simulink model "blending_tank_auto"  (R2020b)
settings: Solver=FixedStepAuto  StartTime=0.0  StopTime=Inf  RelTol=1e-3
PostLoadFcn:
  | slplc.api.loadDataTypes;
InitFcn:
  | T1_InitialValue = FB_TON.InitialValue;
  | T1_InitialValue.PRE = 20000;
  | 
  | C1_InitialValue = FB_CTU.InitialValue;
  | C1_InitialValue.PRE = 3;
StopFcn:
  | clear T1_InitialValue C1_InitialValue;
undefined symbols (not defined in the file): BOOL, DINT, OTL, REAL, slplc
libraries: simulink x3, sldrtlib x1
(part 2 of 15)

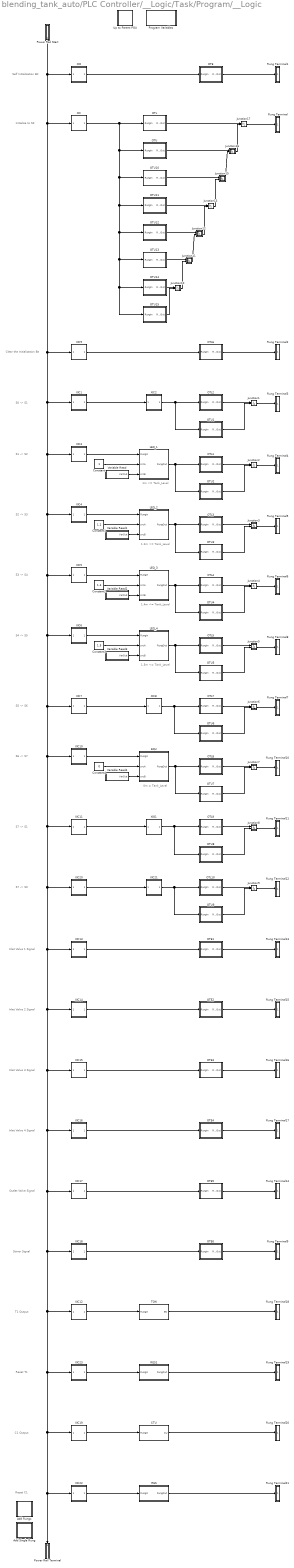
== system blending_tank_auto/PLC Controller/__Logic/Task/Program/__Logic ==
  note: Clear the Initialisation Bit
  note: Self Initialisation Bit
  note: Initialise to S0
  note: S1 -> S2
  note: S0 -> S1
  note: S6 -> S7
  note: S7 -> S1
  note: Inlet Valve 1 Signal
  note: Inlet Valve 2 Signal
  note: Inlet Valve 3 Signal
  note: Inlet Valve 4 Signal
  note: Outlet Valve Signal
  note: Stirrer Signal
  note: S2 -> S3
  note: S3 -> S4
  note: S5 -> S6
  note: S4 -> S5
  note: T1 Output
  note: C1 Output
  note: S7 -> S0
  note: Reset T1
  note: Reset C1
  note: 1m <= Tank_Level
  note: 1.2m <= Tank_Level
  note: 1.4m <= Tank_Level
  note: 1.5m <= Tank_Level
  note: 0m = Tank_Level
  Add Rungs : Subsystem  DisableCoverage=on  TreatAsAtomicUnit=on  mask{PLCRungNumberToAdd=18, PLCBlockType=AddRungs}
      mask prompts: PLCRungNumberToAdd "Rung Number:"
      mask Help: web([docroot '/plccoder/ref/addrungs' '.html']);
      mask DialogControl PLCAddRungs Prompt: Add Rungs
      mask DialogControl PLCRungAddButton Prompt: Add
      mask DialogControl PLCRungAddButton Callback: slplc.callbacks.addLadderRungs(gcb);
      mask Display: disp(sprintf(['Add' newline 'Rungs']));
  Add Single Rung : Subsystem  DisableCoverage=on  TreatAsAtomicUnit=on  mask{PLCRungNumberToAdd=1, PLCBlockType=AddSingleRung}
      settings: OpenFcn=slplc.callbacks.addLadderRungs(gcb);
      mask Help: web([docroot '/plccoder/ref/addsinglerung' '.html']);
      mask DialogControl PLCAddRung Prompt: Add Single Rung
      mask Display: disp(sprintf(['Add' newline '1 Rung']));
  CTU : Subsystem  Priority=114  TreatAsAtomicUnit=on  mask{PLCOperandTag=C1, PLCBlockType=CTU, PLCPOUType=stdFB, PLCOperandAccess=ReadWrite, PLCOperandExpression=xxx_PLC_VAR_C1}
      mask prompts: PLCOperandTag "Counter Tag:"
      mask init:
      | block = gcb;
      | maskObj = Simulink.Mask.get(block);
      | maskObj.Display = sprintf('disp([''%s'' newline newline ''%s'']);', 'CTU', PLCOperandTag);
      | slplc.callbacks.initInstruction(block);
      settings: AttributesFormatString=%<PLCBlockType>: %<PLCOperandTag>
      mask Help: web([docroot '/plccoder/ref/ctu' '.html']);
      mask DialogControl PLCBlockTitle Prompt: Count Up (CTU)
      mask Display: disp(['CTU' newline newline 'C1']);
  Constant : Constant  Priority=32  OutDataTypeStr=double
  Constant1 : Constant  Priority=40  Value=1.2  OutDataTypeStr=double
  Constant2 : Constant  Priority=48  Value=1.4  OutDataTypeStr=double
  Constant3 : Constant  Priority=56  Value=1.5  OutDataTypeStr=double
  Constant4 : Constant  Priority=70  Value=0  OutDataTypeStr=double
  EQU : Subsystem  Priority=72  TreatAsAtomicUnit=on  mask{PLCBlockType=EQU, PLCPOUType=stdFC}
      mask Help: web([docroot '/plccoder/ref/equ' '.html']);
      mask DialogControl PLCBlockTitle Prompt: Equal To (EQU)
      mask DialogControl PLCBlockDesc Prompt: Test whether Source A is equal to Source B.
      mask Display: disp('EQU');
  Junction1 : Subsystem  Priority=29  DisableCoverage=on  TreatAsAtomicUnit=on  mask{PLCBlockType=Junction, PLCPOUType=BranchJunction}
      mask Help: web([docroot '/plccoder/ref/junction' '.html']);
      mask DialogControl PLCBlockTitle Prompt: Rung Merge Point
      mask DialogControl PLCBlockDesc Prompt: This is the ladder diagram rung merge point.
  Junction10 : Subsystem  Priority=14  DisableCoverage=on  TreatAsAtomicUnit=on  mask{PLCBlockType=Junction, PLCPOUType=BranchJunction}
      mask Help: web([docroot '/plccoder/ref/junction' '.html']);
      mask DialogControl PLCBlockTitle Prompt: Rung Merge Point
      mask DialogControl PLCBlockDesc Prompt: This is the ladder diagram rung merge point.
  Junction11 : Subsystem  Priority=15  DisableCoverage=on  TreatAsAtomicUnit=on  mask{PLCBlockType=Junction, PLCPOUType=BranchJunction}
      mask Help: web([docroot '/plccoder/ref/junction' '.html']);
      mask DialogControl PLCBlockTitle Prompt: Rung Merge Point
      mask DialogControl PLCBlockDesc Prompt: This is the ladder diagram rung merge point.
  Junction12 : Subsystem  Priority=16  DisableCoverage=on  TreatAsAtomicUnit=on  mask{PLCBlockType=Junction, PLCPOUType=BranchJunction}
      mask Help: web([docroot '/plccoder/ref/junction' '.html']);
      mask DialogControl PLCBlockTitle Prompt: Rung Merge Point
      mask DialogControl PLCBlockDesc Prompt: This is the ladder diagram rung merge point.
  Junction13 : Subsystem  Priority=17  DisableCoverage=on  TreatAsAtomicUnit=on  mask{PLCBlockType=Junction, PLCPOUType=BranchJunction}
      mask Help: web([docroot '/plccoder/ref/junction' '.html']);
      mask DialogControl PLCBlockTitle Prompt: Rung Merge Point
      mask DialogControl PLCBlockDesc Prompt: This is the ladder diagram rung merge point.
  Junction15 : Subsystem  Priority=18  DisableCoverage=on  TreatAsAtomicUnit=on  mask{PLCBlockType=Junction, PLCPOUType=BranchJunction}
      mask Help: web([docroot '/plccoder/ref/junction' '.html']);
      mask DialogControl PLCBlockTitle Prompt: Rung Merge Point
      mask DialogControl PLCBlockDesc Prompt: This is the ladder diagram rung merge point.
  Junction16 : Subsystem  Priority=19  DisableCoverage=on  TreatAsAtomicUnit=on  mask{PLCBlockType=Junction, PLCPOUType=BranchJunction}
      mask Help: web([docroot '/plccoder/ref/junction' '.html']);
      mask DialogControl PLCBlockTitle Prompt: Rung Merge Point
      mask DialogControl PLCBlockDesc Prompt: This is the ladder diagram rung merge point.
  Junction17 : Subsystem  Priority=20  DisableCoverage=on  TreatAsAtomicUnit=on  mask{PLCBlockType=Junction, PLCPOUType=BranchJunction}
      mask Help: web([docroot '/plccoder/ref/junction' '.html']);
      mask DialogControl PLCBlockTitle Prompt: Rung Merge Point
      mask DialogControl PLCBlockDesc Prompt: This is the ladder diagram rung merge point.
  Junction2 : Subsystem  Priority=37  DisableCoverage=on  TreatAsAtomicUnit=on  mask{PLCBlockType=Junction, PLCPOUType=BranchJunction}
      mask Help: web([docroot '/plccoder/ref/junction' '.html']);
      mask DialogControl PLCBlockTitle Prompt: Rung Merge Point
      mask DialogControl PLCBlockDesc Prompt: This is the ladder diagram rung merge point.
  Junction3 : Subsystem  Priority=45  DisableCoverage=on  TreatAsAtomicUnit=on  mask{PLCBlockType=Junction, PLCPOUType=BranchJunction}
      mask Help: web([docroot '/plccoder/ref/junction' '.html']);
      mask DialogControl PLCBlockTitle Prompt: Rung Merge Point
      mask DialogControl PLCBlockDesc Prompt: This is the ladder diagram rung merge point.
  Junction4 : Subsystem  Priority=53  DisableCoverage=on  TreatAsAtomicUnit=on  mask{PLCBlockType=Junction, PLCPOUType=BranchJunction}
      mask Help: web([docroot '/plccoder/ref/junction' '.html']);
      mask DialogControl PLCBlockTitle Prompt: Rung Merge Point
      mask DialogControl PLCBlockDesc Prompt: This is the ladder diagram rung merge point.
  Junction5 : Subsystem  Priority=61  DisableCoverage=on  TreatAsAtomicUnit=on  mask{PLCBlockType=Junction, PLCPOUType=BranchJunction}
      mask Help: web([docroot '/plccoder/ref/junction' '.html']);
      mask DialogControl PLCBlockTitle Prompt: Rung Merge Point
      mask DialogControl PLCBlockDesc Prompt: This is the ladder diagram rung merge point.
  Junction6 : Subsystem  Priority=67  DisableCoverage=on  TreatAsAtomicUnit=on  mask{PLCBlockType=Junction, PLCPOUType=BranchJunction}
      mask Help: web([docroot '/plccoder/ref/junction' '.html']);
      mask DialogControl PLCBlockTitle Prompt: Rung Merge Point
      mask DialogControl PLCBlockDesc Prompt: This is the ladder diagram rung merge point.
  Junction7 : Subsystem  Priority=75  DisableCoverage=on  TreatAsAtomicUnit=on  mask{PLCBlockType=Junction, PLCPOUType=BranchJunction}
      mask Help: web([docroot '/plccoder/ref/junction' '.html']);
      mask DialogControl PLCBlockTitle Prompt: Rung Merge Point
      mask DialogControl PLCBlockDesc Prompt: This is the ladder diagram rung merge point.
  Junction8 : Subsystem  Priority=81  DisableCoverage=on  TreatAsAtomicUnit=on  mask{PLCBlockType=Junction, PLCPOUType=BranchJunction}
      mask Help: web([docroot '/plccoder/ref/junction' '.html']);
      mask DialogControl PLCBlockTitle Prompt: Rung Merge Point
      mask DialogControl PLCBlockDesc Prompt: This is the ladder diagram rung merge point.
  Junction9 : Subsystem  Priority=87  DisableCoverage=on  TreatAsAtomicUnit=on  mask{PLCBlockType=Junction, PLCPOUType=BranchJunction}
      mask Help: web([docroot '/plccoder/ref/junction' '.html']);
      mask DialogControl PLCBlockTitle Prompt: Rung Merge Point
      mask DialogControl PLCBlockDesc Prompt: This is the ladder diagram rung merge point.
  LEQ_1 : Subsystem  Priority=34  TreatAsAtomicUnit=on  mask{PLCBlockType=LEQ, PLCPOUType=stdFC}
      mask Help: web([docroot '/plccoder/ref/leq' '.html']);
      mask DialogControl PLCBlockTitle Prompt: Less Than or Equal To (LEQ)
      mask DialogControl PLCBlockDesc Prompt: Test whether Source A is less than or equal to Source B.
      mask Display: disp('LEQ');
  LEQ_2 : Subsystem  Priority=42  TreatAsAtomicUnit=on  mask{PLCBlockType=LEQ, PLCPOUType=stdFC}
      mask Help: web([docroot '/plccoder/ref/leq' '.html']);
      mask DialogControl PLCBlockTitle Prompt: Less Than or Equal To (LEQ)
      mask DialogControl PLCBlockDesc Prompt: Test whether Source A is less than or equal to Source B.
      mask Display: disp('LEQ');
  LEQ_3 : Subsystem  Priority=50  TreatAsAtomicUnit=on  mask{PLCBlockType=LEQ, PLCPOUType=stdFC}
      mask Help: web([docroot '/plccoder/ref/leq' '.html']);
      mask DialogControl PLCBlockTitle Prompt: Less Than or Equal To (LEQ)
      mask DialogControl PLCBlockDesc Prompt: Test whether Source A is less than or equal to Source B.
      mask Display: disp('LEQ');
  LEQ_4 : Subsystem  Priority=58  TreatAsAtomicUnit=on  mask{PLCBlockType=LEQ, PLCPOUType=stdFC}
      mask Help: web([docroot '/plccoder/ref/leq' '.html']);
      mask DialogControl PLCBlockTitle Prompt: Less Than or Equal To (LEQ)
      mask DialogControl PLCBlockDesc Prompt: Test whether Source A is less than or equal to Source B.
      mask Display: disp('LEQ');
  OTE : Subsystem  Priority=3  TreatAsAtomicUnit=on  mask{PLCOperandTag=Initialise, PLCBlockType=OTE, PLCPOUType=Coil, PLCOperandExpression=xxx_PLC_VAR_Initialise}
      mask prompts: PLCOperandTag "Operand Tag:"
      mask init:
      | slplc.callbacks.initInstruction(gcb);
      settings: AttributesFormatString=%<PLCOperandTag>
      mask Help: web([docroot '/plccoder/ref/ote' '.html']);
      mask DialogControl PLCBlockTitle Prompt: Output Energize (OTE)
  OTE1 : Subsystem  Priority=90  TreatAsAtomicUnit=on  mask{PLCOperandTag=IV1_Signal, PLCBlockType=OTE, PLCPOUType=Coil, PLCOperandExpression=xxx_PLC_VAR_IV1_Signal}
      mask prompts: PLCOperandTag "Operand Tag:"
      mask init:
      | slplc.callbacks.initInstruction(gcb);
      settings: AttributesFormatString=%<PLCOperandTag>
      mask Help: web([docroot '/plccoder/ref/ote' '.html']);
      mask DialogControl PLCBlockTitle Prompt: Output Energize (OTE)
  OTE2 : Subsystem  Priority=93  TreatAsAtomicUnit=on  mask{PLCOperandTag=IV2_Signal, PLCBlockType=OTE, PLCPOUType=Coil, PLCOperandExpression=xxx_PLC_VAR_IV2_Signal}
      mask prompts: PLCOperandTag "Operand Tag:"
      mask init:
      | slplc.callbacks.initInstruction(gcb);
      settings: AttributesFormatString=%<PLCOperandTag>
      mask Help: web([docroot '/plccoder/ref/ote' '.html']);
      mask DialogControl PLCBlockTitle Prompt: Output Energize (OTE)
  OTE3 : Subsystem  Priority=96  TreatAsAtomicUnit=on  mask{PLCOperandTag=IV3_Signal, PLCBlockType=OTE, PLCPOUType=Coil, PLCOperandExpression=xxx_PLC_VAR_IV3_Signal}
      mask prompts: PLCOperandTag "Operand Tag:"
      mask init:
      | slplc.callbacks.initInstruction(gcb);
      settings: AttributesFormatString=%<PLCOperandTag>
      mask Help: web([docroot '/plccoder/ref/ote' '.html']);
      mask DialogControl PLCBlockTitle Prompt: Output Energize (OTE)
  OTE4 : Subsystem  Priority=99  TreatAsAtomicUnit=on  mask{PLCOperandTag=IV4_Signal, PLCBlockType=OTE, PLCPOUType=Coil, PLCOperandExpression=xxx_PLC_VAR_IV4_Signal}
      mask prompts: PLCOperandTag "Operand Tag:"
      mask init:
      | slplc.callbacks.initInstruction(gcb);
      settings: AttributesFormatString=%<PLCOperandTag>
      mask Help: web([docroot '/plccoder/ref/ote' '.html']);
      mask DialogControl PLCBlockTitle Prompt: Output Energize (OTE)
  OTE5 : Subsystem  Priority=102  TreatAsAtomicUnit=on  mask{PLCOperandTag=OV_Signal, PLCBlockType=OTE, PLCPOUType=Coil, PLCOperandExpression=xxx_PLC_VAR_OV_Signal}
      mask prompts: PLCOperandTag "Operand Tag:"
      mask init:
      | slplc.callbacks.initInstruction(gcb);
      settings: AttributesFormatString=%<PLCOperandTag>
      mask Help: web([docroot '/plccoder/ref/ote' '.html']);
      mask DialogControl PLCBlockTitle Prompt: Output Energize (OTE)
  OTE6 : Subsystem  Priority=105  TreatAsAtomicUnit=on  mask{PLCOperandTag=Stirrer_Signal, PLCBlockType=OTE, PLCPOUType=Coil, PLCOperandExpression=xxx_PLC_VAR_Stirrer_Signal}
      mask prompts: PLCOperandTag "Operand Tag:"
      mask init:
      | slplc.callbacks.initInstruction(gcb);
      settings: AttributesFormatString=%<PLCOperandTag>
      mask Help: web([docroot '/plccoder/ref/ote' '.html']);
      mask DialogControl PLCBlockTitle Prompt: Output Energize (OTE)
  OTL : Subsystem  Priority=6  TreatAsAtomicUnit=on  mask{PLCOperandTag=M0, PLCBlockType=OTL, PLCPOUType=Coil, PLCOperandExpression=xxx_PLC_VAR_M0}
      mask prompts: PLCOperandTag "Operand Tag:"
      mask init:
      | slplc.callbacks.initInstruction(gcb);
      settings: AttributesFormatString=%<PLCOperandTag>
      mask Help: web([docroot '/plccoder/ref/otl' '.html']);
      mask DialogControl PLCBlockTitle Prompt: Output Latch (OTL)
      mask Display: disp('L');
  OTL1 : Subsystem  Priority=35  TreatAsAtomicUnit=on  mask{PLCOperandTag=M2, PLCBlockType=OTL, PLCPOUType=Coil, PLCOperandExpression=xxx_PLC_VAR_M2}
      mask prompts: PLCOperandTag "Operand Tag:"
      mask init:
      | slplc.callbacks.initInstruction(gcb);
      settings: AttributesFormatString=%<PLCOperandTag>
      mask Help: web([docroot '/plccoder/ref/otl' '.html']);
      mask DialogControl PLCBlockTitle Prompt: Output Latch (OTL)
      mask Display: disp('L');
  OTL10 : Subsystem  Priority=85  TreatAsAtomicUnit=on  mask{PLCOperandTag=M0, PLCBlockType=OTL, PLCPOUType=Coil, PLCOperandExpression=xxx_PLC_VAR_M0}
      mask prompts: PLCOperandTag "Operand Tag:"
      mask init:
      | slplc.callbacks.initInstruction(gcb);
      settings: AttributesFormatString=%<PLCOperandTag>
      mask Help: web([docroot '/plccoder/ref/otl' '.html']);
      mask DialogControl PLCBlockTitle Prompt: Output Latch (OTL)
      mask Display: disp('L');
  OTL2 : Subsystem  Priority=27  TreatAsAtomicUnit=on  mask{PLCOperandTag=M1, PLCBlockType=OTL, PLCPOUType=Coil, PLCOperandExpression=xxx_PLC_VAR_M1}
      mask prompts: PLCOperandTag "Operand Tag:"
      mask init:
      | slplc.callbacks.initInstruction(gcb);
      settings: AttributesFormatString=%<PLCOperandTag>
      mask Help: web([docroot '/plccoder/ref/otl' '.html']);
      mask DialogControl PLCBlockTitle Prompt: Output Latch (OTL)
      mask Display: disp('L');
  OTL3 : Subsystem  Priority=43  TreatAsAtomicUnit=on  mask{PLCOperandTag=M3, PLCBlockType=OTL, PLCPOUType=Coil, PLCOperandExpression=xxx_PLC_VAR_M3}
      mask prompts: PLCOperandTag "Operand Tag:"
      mask init:
      | slplc.callbacks.initInstruction(gcb);
      settings: AttributesFormatString=%<PLCOperandTag>
      mask Help: web([docroot '/plccoder/ref/otl' '.html']);
      mask DialogControl PLCBlockTitle Prompt: Output Latch (OTL)
      mask Display: disp('L');
  OTL4 : Subsystem  Priority=51  TreatAsAtomicUnit=on  mask{PLCOperandTag=M4, PLCBlockType=OTL, PLCPOUType=Coil, PLCOperandExpression=xxx_PLC_VAR_M4}
      mask prompts: PLCOperandTag "Operand Tag:"
      mask init:
      | slplc.callbacks.initInstruction(gcb);
      settings: AttributesFormatString=%<PLCOperandTag>
      mask Help: web([docroot '/plccoder/ref/otl' '.html']);
      mask DialogControl PLCBlockTitle Prompt: Output Latch (OTL)
      mask Display: disp('L');
  OTL5 : Subsystem  Priority=59  TreatAsAtomicUnit=on  mask{PLCOperandTag=M5, PLCBlockType=OTL, PLCPOUType=Coil, PLCOperandExpression=xxx_PLC_VAR_M5}
      mask prompts: PLCOperandTag "Operand Tag:"
      mask init:
      | slplc.callbacks.initInstruction(gcb);
      settings: AttributesFormatString=%<PLCOperandTag>
      mask Help: web([docroot '/plccoder/ref/otl' '.html']);
      mask DialogControl PLCBlockTitle Prompt: Output Latch (OTL)
      mask Display: disp('L');
  OTL6 : Subsystem  Priority=23  TreatAsAtomicUnit=on  mask{PLCOperandTag=Running, PLCBlockType=OTL, PLCPOUType=Coil, PLCOperandExpression=xxx_PLC_VAR_Running}
      mask prompts: PLCOperandTag "Operand Tag:"
      mask init:
      | slplc.callbacks.initInstruction(gcb);
      settings: AttributesFormatString=%<PLCOperandTag>
      mask Help: web([docroot '/plccoder/ref/otl' '.html']);
      mask DialogControl PLCBlockTitle Prompt: Output Latch (OTL)
      mask Display: disp('L');
  OTL7 : Subsystem  Priority=65  TreatAsAtomicUnit=on  mask{PLCOperandTag=M6, PLCBlockType=OTL, PLCPOUType=Coil, PLCOperandExpression=xxx_PLC_VAR_M6}
      mask prompts: PLCOperandTag "Operand Tag:"
      mask init:
      | slplc.callbacks.initInstruction(gcb);
      settings: AttributesFormatString=%<PLCOperandTag>
      mask Help: web([docroot '/plccoder/ref/otl' '.html']);
      mask DialogControl PLCBlockTitle Prompt: Output Latch (OTL)
      mask Display: disp('L');
  OTL8 : Subsystem  Priority=73  TreatAsAtomicUnit=on  mask{PLCOperandTag=M7, PLCBlockType=OTL, PLCPOUType=Coil, PLCOperandExpression=xxx_PLC_VAR_M7}
      mask prompts: PLCOperandTag "Operand Tag:"
      mask init:
      | slplc.callbacks.initInstruction(gcb);
      settings: AttributesFormatString=%<PLCOperandTag>
      mask Help: web([docroot '/plccoder/ref/otl' '.html']);
      mask DialogControl PLCBlockTitle Prompt: Output Latch (OTL)
      mask Display: disp('L');
  OTL9 : Subsystem  Priority=79  TreatAsAtomicUnit=on  mask{PLCOperandTag=M1, PLCBlockType=OTL, PLCPOUType=Coil, PLCOperandExpression=xxx_PLC_VAR_M1}
      mask prompts: PLCOperandTag "Operand Tag:"
      mask init:
      | slplc.callbacks.initInstruction(gcb);
      settings: AttributesFormatString=%<PLCOperandTag>
      mask Help: web([docroot '/plccoder/ref/otl' '.html']);
      mask DialogControl PLCBlockTitle Prompt: Output Latch (OTL)
      mask Display: disp('L');
  OTU : Subsystem  Priority=7  TreatAsAtomicUnit=on  mask{PLCOperandTag=M1, PLCBlockType=OTU, PLCPOUType=Coil, PLCOperandExpression=xxx_PLC_VAR_M1}
      mask prompts: PLCOperandTag "Operand Tag:"
      mask init:
      | slplc.callbacks.initInstruction(gcb);
      settings: AttributesFormatString=%<PLCOperandTag>
      mask Help: web([docroot '/plccoder/ref/otu' '.html']);
      mask DialogControl PLCBlockTitle Prompt: Output Unlatch (OTU)
      mask Display: disp('U');
  OTU1 : Subsystem  Priority=28  TreatAsAtomicUnit=on  mask{PLCOperandTag=M0, PLCBlockType=OTU, PLCPOUType=Coil, PLCOperandExpression=xxx_PLC_VAR_M0}
      mask prompts: PLCOperandTag "Operand Tag:"
      mask init:
      | slplc.callbacks.initInstruction(gcb);
      settings: AttributesFormatString=%<PLCOperandTag>
      mask Help: web([docroot '/plccoder/ref/otu' '.html']);
      mask DialogControl PLCBlockTitle Prompt: Output Unlatch (OTU)
      mask Display: disp('U');
  OTU10 : Subsystem  Priority=8  TreatAsAtomicUnit=on  mask{PLCOperandTag=M2, PLCBlockType=OTU, PLCPOUType=Coil, PLCOperandExpression=xxx_PLC_VAR_M2}
      mask prompts: PLCOperandTag "Operand Tag:"
      mask init:
      | slplc.callbacks.initInstruction(gcb);
      settings: AttributesFormatString=%<PLCOperandTag>
      mask Help: web([docroot '/plccoder/ref/otu' '.html']);
      mask DialogControl PLCBlockTitle Prompt: Output Unlatch (OTU)
      mask Display: disp('U');
  OTU11 : Subsystem  Priority=9  TreatAsAtomicUnit=on  mask{PLCOperandTag=M3, PLCBlockType=OTU, PLCPOUType=Coil, PLCOperandExpression=xxx_PLC_VAR_M3}
      mask prompts: PLCOperandTag "Operand Tag:"
      mask init:
      | slplc.callbacks.initInstruction(gcb);
      settings: AttributesFormatString=%<PLCOperandTag>
      mask Help: web([docroot '/plccoder/ref/otu' '.html']);
      mask DialogControl PLCBlockTitle Prompt: Output Unlatch (OTU)
      mask Display: disp('U');
  OTU12 : Subsystem  Priority=10  TreatAsAtomicUnit=on  mask{PLCOperandTag=M4, PLCBlockType=OTU, PLCPOUType=Coil, PLCOperandExpression=xxx_PLC_VAR_M4}
      mask prompts: PLCOperandTag "Operand Tag:"
      mask init:
      | slplc.callbacks.initInstruction(gcb);
      settings: AttributesFormatString=%<PLCOperandTag>
      mask Help: web([docroot '/plccoder/ref/otu' '.html']);
      mask DialogControl PLCBlockTitle Prompt: Output Unlatch (OTU)
      mask Display: disp('U');
  OTU13 : Subsystem  Priority=11  TreatAsAtomicUnit=on  mask{PLCOperandTag=M5, PLCBlockType=OTU, PLCPOUType=Coil, PLCOperandExpression=xxx_PLC_VAR_M5}
      mask prompts: PLCOperandTag "Operand Tag:"
      mask init:
      | slplc.callbacks.initInstruction(gcb);
      settings: AttributesFormatString=%<PLCOperandTag>
      mask Help: web([docroot '/plccoder/ref/otu' '.html']);
      mask DialogControl PLCBlockTitle Prompt: Output Unlatch (OTU)
      mask Display: disp('U');
  OTU14 : Subsystem  Priority=12  TreatAsAtomicUnit=on  mask{PLCOperandTag=M6, PLCBlockType=OTU, PLCPOUType=Coil, PLCOperandExpression=xxx_PLC_VAR_M6}
      mask prompts: PLCOperandTag "Operand Tag:"
      mask init:
      | slplc.callbacks.initInstruction(gcb);
      settings: AttributesFormatString=%<PLCOperandTag>
      mask Help: web([docroot '/plccoder/ref/otu' '.html']);
      mask DialogControl PLCBlockTitle Prompt: Output Unlatch (OTU)
      mask Display: disp('U');
  OTU15 : Subsystem  Priority=13  TreatAsAtomicUnit=on  mask{PLCOperandTag=M7, PLCBlockType=OTU, PLCPOUType=Coil, PLCOperandExpression=xxx_PLC_VAR_M7}
      mask prompts: PLCOperandTag "Operand Tag:"
      mask init:
      | slplc.callbacks.initInstruction(gcb);
      settings: AttributesFormatString=%<PLCOperandTag>
      mask Help: web([docroot '/plccoder/ref/otu' '.html']);
      mask DialogControl PLCBlockTitle Prompt: Output Unlatch (OTU)
      mask Display: disp('U');
  OTU2 : Subsystem  Priority=36  TreatAsAtomicUnit=on  mask{PLCOperandTag=M1, PLCBlockType=OTU, PLCPOUType=Coil, PLCOperandExpression=xxx_PLC_VAR_M1}
      mask prompts: PLCOperandTag "Operand Tag:"
      mask init:
      | slplc.callbacks.initInstruction(gcb);
      settings: AttributesFormatString=%<PLCOperandTag>
      mask Help: web([docroot '/plccoder/ref/otu' '.html']);
      mask DialogControl PLCBlockTitle Prompt: Output Unlatch (OTU)
      mask Display: disp('U');
  OTU3 : Subsystem  Priority=44  TreatAsAtomicUnit=on  mask{PLCOperandTag=M2, PLCBlockType=OTU, PLCPOUType=Coil, PLCOperandExpression=xxx_PLC_VAR_M2}
      mask prompts: PLCOperandTag "Operand Tag:"
      mask init:
      | slplc.callbacks.initInstruction(gcb);
      settings: AttributesFormatString=%<PLCOperandTag>
      mask Help: web([docroot '/plccoder/ref/otu' '.html']);
      mask DialogControl PLCBlockTitle Prompt: Output Unlatch (OTU)
      mask Display: disp('U');
  OTU4 : Subsystem  Priority=52  TreatAsAtomicUnit=on  mask{PLCOperandTag=M3, PLCBlockType=OTU, PLCPOUType=Coil, PLCOperandExpression=xxx_PLC_VAR_M3}
      mask prompts: PLCOperandTag "Operand Tag:"
      mask init:
      | slplc.callbacks.initInstruction(gcb);
      settings: AttributesFormatString=%<PLCOperandTag>
      mask Help: web([docroot '/plccoder/ref/otu' '.html']);
      mask DialogControl PLCBlockTitle Prompt: Output Unlatch (OTU)
      mask Display: disp('U');
  OTU5 : Subsystem  Priority=60  TreatAsAtomicUnit=on  mask{PLCOperandTag=M4, PLCBlockType=OTU, PLCPOUType=Coil, PLCOperandExpression=xxx_PLC_VAR_M4}
      mask prompts: PLCOperandTag "Operand Tag:"
      mask init:
      | slplc.callbacks.initInstruction(gcb);
      settings: AttributesFormatString=%<PLCOperandTag>
      mask Help: web([docroot '/plccoder/ref/otu' '.html']);
      mask DialogControl PLCBlockTitle Prompt: Output Unlatch (OTU)
      mask Display: disp('U');
  OTU6 : Subsystem  Priority=66  TreatAsAtomicUnit=on  mask{PLCOperandTag=M5, PLCBlockType=OTU, PLCPOUType=Coil, PLCOperandExpression=xxx_PLC_VAR_M5}
      mask prompts: PLCOperandTag "Operand Tag:"
      mask init:
      | slplc.callbacks.initInstruction(gcb);
      settings: AttributesFormatString=%<PLCOperandTag>
      mask Help: web([docroot '/plccoder/ref/otu' '.html']);
      mask DialogControl PLCBlockTitle Prompt: Output Unlatch (OTU)
      mask Display: disp('U');
  OTU7 : Subsystem  Priority=74  TreatAsAtomicUnit=on  mask{PLCOperandTag=M6, PLCBlockType=OTU, PLCPOUType=Coil, PLCOperandExpression=xxx_PLC_VAR_M6}
      mask prompts: PLCOperandTag "Operand Tag:"
      mask init:
      | slplc.callbacks.initInstruction(gcb);
      settings: AttributesFormatString=%<PLCOperandTag>
      mask Help: web([docroot '/plccoder/ref/otu' '.html']);
      mask DialogControl PLCBlockTitle Prompt: Output Unlatch (OTU)
      mask Display: disp('U');
  OTU8 : Subsystem  Priority=80  TreatAsAtomicUnit=on  mask{PLCOperandTag=M7, PLCBlockType=OTU, PLCPOUType=Coil, PLCOperandExpression=xxx_PLC_VAR_M7}
      mask prompts: PLCOperandTag "Operand Tag:"
      mask init:
      | slplc.callbacks.initInstruction(gcb);
      settings: AttributesFormatString=%<PLCOperandTag>
      mask Help: web([docroot '/plccoder/ref/otu' '.html']);
      mask DialogControl PLCBlockTitle Prompt: Output Unlatch (OTU)
      mask Display: disp('U');
  OTU9 : Subsystem  Priority=86  TreatAsAtomicUnit=on  mask{PLCOperandTag=M7, PLCBlockType=OTU, PLCPOUType=Coil, PLCOperandExpression=xxx_PLC_VAR_M7}
      mask prompts: PLCOperandTag "Operand Tag:"
      mask init:
      | slplc.callbacks.initInstruction(gcb);
      settings: AttributesFormatString=%<PLCOperandTag>
      mask Help: web([docroot '/plccoder/ref/otu' '.html']);
      mask DialogControl PLCBlockTitle Prompt: Output Unlatch (OTU)
      mask Display: disp('U');
  Power Rail Start : Subsystem  Priority=1  DisableCoverage=on  TreatAsAtomicUnit=on  mask{PLCBlockType=PowerRailStart}
      mask Help: web([docroot '/plccoder/ref/powerrailstart' '.html']);
      mask DialogControl PLCBlockTitle Prompt: Power Rail Start
      mask DialogControl PLCBlockDesc Prompt: This is the ladder diagram left power rail start block.
  Power Rail Terminal : Subsystem  DisableCoverage=on  TreatAsAtomicUnit=on  mask{PLCBlockType=PowerRailTerminal}
      mask Help: web([docroot '/plccoder/ref/powerrailterminal' '.html']);
      mask DialogControl PLCBlockTitle Prompt: Power Rail Terminal
      mask DialogControl PLCBlockDesc Prompt: This is the ladder diagram left power rail terminal block.
  Program Variables : Subsystem  Tag=ProgramVariableSS  DisableCoverage=on  TreatAsAtomicUnit=on  mask{PLCVarC1Name=C1, PLCVarC1Scope=Local, PLCVarC1PortType=Hidden, PLCVarC1PortIndex=20, PLCVarC1DataType=Bus: COUNTER, PLCVarC1Size=1, PLCVarC1InitialValue=C1_InitialValue, PLCVarC1ToDelete=off, PLCVarInitialiseName=Initialise, PLCVarInitialiseScope=Local, PLCVarInitialisePortType=Hidden, PLCVarInitialisePortIndex=20, PLCVarInitialiseDataType=BOOL, PLCVarInitialiseSize=1, PLCVarInitialiseInitialValue=false, PLCVarInitialiseToDelete=off, PLCVarM0Name=M0, PLCVarM0Scope=Local, PLCVarM0PortType=Hidden, PLCVarM0PortIndex=20, PLCVarM0DataType=BOOL, PLCVarM0Size=1, PLCVarM0InitialValue=false, PLCVarM0ToDelete=off, PLCVarM1Name=M1, PLCVarM1Scope=Local, PLCVarM1PortType=Hidden, PLCVarM1PortIndex=20, PLCVarM1DataType=BOOL, PLCVarM1Size=1, PLCVarM1InitialValue=false, PLCVarM1ToDelete=off, PLCVarM2Name=M2, PLCVarM2Scope=Local, PLCVarM2PortType=Hidden, PLCVarM2PortIndex=20, PLCVarM2DataType=BOOL, PLCVarM2Size=1, PLCVarM2InitialValue=false, PLCVarM2ToDelete=off, PLCVarM3Name=M3, PLCVarM3Scope=Local, PLCVarM3PortType=Hidden, PLCVarM3PortIndex=20, PLCVarM3DataType=BOOL, PLCVarM3Size=1, PLCVarM3InitialValue=false, PLCVarM3ToDelete=off, PLCVarM4Name=M4, PLCVarM4Scope=Local, PLCVarM4PortType=Hidden, PLCVarM4PortIndex=20, PLCVarM4DataType=BOOL, PLCVarM4Size=1, PLCVarM4InitialValue=false, PLCVarM4ToDelete=off, PLCVarM5Name=M5, PLCVarM5Scope=Local, PLCVarM5PortType=Hidden, PLCVarM5PortIndex=20, PLCVarM5DataType=BOOL, PLCVarM5Size=1, PLCVarM5InitialValue=false, PLCVarM5ToDelete=off, PLCVarM6Name=M6, PLCVarM6Scope=Local, PLCVarM6PortType=Hidden, PLCVarM6PortIndex=20, PLCVarM6DataType=BOOL, PLCVarM6Size=1, PLCVarM6InitialValue=false, PLCVarM6ToDelete=off, PLCVarM7Name=M7, PLCVarM7Scope=Local, PLCVarM7PortType=Hidden, PLCVarM7PortIndex=20, PLCVarM7DataType=BOOL, PLCVarM7Size=1, PLCVarM7InitialValue=false, PLCVarM7ToDelete=off, PLCVarRunningName=Running, PLCVarRunningScope=Local, PLCVarRunningPortType=Hidden, PLCVarRunningPortIndex=20, PLCVarRunningDataType=BOOL, PLCVarRunningSize=1, PLCVarRunningInitialValue=false, PLCVarRunningToDelete=off, PLCVarT1Name=T1, PLCVarT1Scope=Local, PLCVarT1PortType=Hidden, PLCVarT1PortIndex=20, PLCVarT1DataType=Bus: TIMER, PLCVarT1Size=1, PLCVarT1InitialValue=T1_InitialValue, PLCVarT1ToDelete=off, PLCVarIV1_SignalName=IV1_Signal, PLCVarIV1_SignalScope=External, PLCVarIV1_SignalPortType=Hidden, PLCVarIV1_SignalPortIndex=20, PLCVarIV1_SignalDataType=DINT, PLCVarIV1_SignalSize=-1, PLCVarIV1_SignalInitialValue=0, PLCVarIV1_SignalToDelete=off, PLCVarIV2_SignalName=IV2_Signal, PLCVarIV2_SignalScope=External, PLCVarIV2_SignalPortType=Hidden, PLCVarIV2_SignalPortIndex=20, PLCVarIV2_SignalDataType=DINT, PLCVarIV2_SignalSize=-1, PLCVarIV2_SignalInitialValue=0, PLCVarIV2_SignalToDelete=off, PLCVarIV3_SignalName=IV3_Signal, PLCVarIV3_SignalScope=External, PLCVarIV3_SignalPortType=Hidden, PLCVarIV3_SignalPortIndex=20, PLCVarIV3_SignalDataType=DINT, PLCVarIV3_SignalSize=-1, PLCVarIV3_SignalInitialValue=0, PLCVarIV3_SignalToDelete=off, PLCVarIV4_SignalName=IV4_Signal, PLCVarIV4_SignalScope=External, PLCVarIV4_SignalPortType=Hidden, PLCVarIV4_SignalPortIndex=20, PLCVarIV4_SignalDataType=DINT, PLCVarIV4_SignalSize=-1, PLCVarIV4_SignalInitialValue=0, PLCVarIV4_SignalToDelete=off, PLCVarOV_SignalName=OV_Signal, PLCVarOV_SignalScope=External, PLCVarOV_SignalPortType=Hidden, PLCVarOV_SignalPortIndex=20, PLCVarOV_SignalDataType=DINT, PLCVarOV_SignalSize=-1, PLCVarOV_SignalInitialValue=0, PLCVarOV_SignalToDelete=off, PLCVarStart_ButtonName=Start_Button, PLCVarStart_ButtonScope=External, PLCVarStart_ButtonPortType=Hidden, PLCVarStart_ButtonPortIndex=20, PLCVarStart_ButtonDataType=DINT, PLCVarStart_ButtonSize=-1, PLCVarStart_ButtonInitialValue=0, PLCVarStart_ButtonToDelete=off, PLCVarStirrer_SignalName=Stirrer_Signal, PLCVarStirrer_SignalScope=External, PLCVarStirrer_SignalPortType=Hidden, PLCVarStirrer_SignalPortIndex=20, PLCVarStirrer_SignalDataType=DINT, PLCVarStirrer_SignalSize=-1, PLCVarStirrer_SignalInitialValue=0, PLCVarStirrer_SignalToDelete=off, PLCVarTank_LevelName=Tank_Level, PLCVarTank_LevelScope=External, PLCVarTank_LevelPortType=Hidden, PLCVarTank_LevelPortIndex=20, PLCVarTank_LevelDataType=DINT, PLCVarTank_LevelSize=-1, PLCVarTank_LevelInitialValue=0, PLCVarTank_LevelToDelete=off}
      mask init:
      | slplc.callbacks.initPOUVarSS(gcb);
      settings: OpenFcn=slplc.callbacks.openProgramVariableSS(gcb);
      mask Help: web([docroot '/plccoder/ref/programvariables' '.html']);
      mask TypeOptions PLCVarC1Scope: Local | External
      mask Callback PLCVarC1Scope: slplc.callbacks.updatePOUVarSS(gcb);
      mask TypeOptions PLCVarC1PortType: Hidden | Inport | Outport
      mask Callback PLCVarC1PortType: slplc.callbacks.updatePOUVarSS(gcb);
      mask TypeOptions PLCVarC1PortIndex: 1 | 2 | 3 | 4 | 5 | 6 | 7 | 8 | 9 | 10 | 11 | 12 | 13 | 14 | 15 | 16 | 17 | 18 | 19 | 20
      mask TypeOptions PLCVarInitialiseScope: Local | External
      mask Callback PLCVarInitialiseScope: slplc.callbacks.updatePOUVarSS(gcb);
      mask TypeOptions PLCVarInitialisePortType: Hidden | Inport | Outport
      mask Callback PLCVarInitialisePortType: slplc.callbacks.updatePOUVarSS(gcb);
      mask TypeOptions PLCVarInitialisePortIndex: 1 | 2 | 3 | 4 | 5 | 6 | 7 | 8 | 9 | 10 | 11 | 12 | 13 | 14 | 15 | 16 | 17 | 18 | 19 | 20
      mask TypeOptions PLCVarM0Scope: Local | External
      mask Callback PLCVarM0Scope: slplc.callbacks.updatePOUVarSS(gcb);
      mask TypeOptions PLCVarM0PortType: Hidden | Inport | Outport
      mask Callback PLCVarM0PortType: slplc.callbacks.updatePOUVarSS(gcb);
      mask TypeOptions PLCVarM0PortIndex: 1 | 2 | 3 | 4 | 5 | 6 | 7 | 8 | 9 | 10 | 11 | 12 | 13 | 14 | 15 | 16 | 17 | 18 | 19 | 20
      mask TypeOptions PLCVarM1Scope: Local | External
      mask Callback PLCVarM1Scope: slplc.callbacks.updatePOUVarSS(gcb);
      mask TypeOptions PLCVarM1PortType: Hidden | Inport | Outport
      mask Callback PLCVarM1PortType: slplc.callbacks.updatePOUVarSS(gcb);
      mask TypeOptions PLCVarM1PortIndex: 1 | 2 | 3 | 4 | 5 | 6 | 7 | 8 | 9 | 10 | 11 | 12 | 13 | 14 | 15 | 16 | 17 | 18 | 19 | 20
      mask TypeOptions PLCVarM2Scope: Local | External
      mask Callback PLCVarM2Scope: slplc.callbacks.updatePOUVarSS(gcb);
      mask TypeOptions PLCVarM2PortType: Hidden | Inport | Outport
      mask Callback PLCVarM2PortType: slplc.callbacks.updatePOUVarSS(gcb);
      mask TypeOptions PLCVarM2PortIndex: 1 | 2 | 3 | 4 | 5 | 6 | 7 | 8 | 9 | 10 | 11 | 12 | 13 | 14 | 15 | 16 | 17 | 18 | 19 | 20
      mask TypeOptions PLCVarM3Scope: Local | External
      mask Callback PLCVarM3Scope: slplc.callbacks.updatePOUVarSS(gcb);
      mask TypeOptions PLCVarM3PortType: Hidden | Inport | Outport
      mask Callback PLCVarM3PortType: slplc.callbacks.updatePOUVarSS(gcb);
      mask TypeOptions PLCVarM3PortIndex: 1 | 2 | 3 | 4 | 5 | 6 | 7 | 8 | 9 | 10 | 11 | 12 | 13 | 14 | 15 | 16 | 17 | 18 | 19 | 20
      mask TypeOptions PLCVarM4Scope: Local | External
      mask Callback PLCVarM4Scope: slplc.callbacks.updatePOUVarSS(gcb);
      mask TypeOptions PLCVarM4PortType: Hidden | Inport | Outport
      mask Callback PLCVarM4PortType: slplc.callbacks.updatePOUVarSS(gcb);
      mask TypeOptions PLCVarM4PortIndex: 1 | 2 | 3 | 4 | 5 | 6 | 7 | 8 | 9 | 10 | 11 | 12 | 13 | 14 | 15 | 16 | 17 | 18 | 19 | 20
      mask TypeOptions PLCVarM5Scope: Local | External
      mask Callback PLCVarM5Scope: slplc.callbacks.updatePOUVarSS(gcb);
      mask TypeOptions PLCVarM5PortType: Hidden | Inport | Outport
      mask Callback PLCVarM5PortType: slplc.callbacks.updatePOUVarSS(gcb);
      mask TypeOptions PLCVarM5PortIndex: 1 | 2 | 3 | 4 | 5 | 6 | 7 | 8 | 9 | 10 | 11 | 12 | 13 | 14 | 15 | 16 | 17 | 18 | 19 | 20
      mask TypeOptions PLCVarM6Scope: Local | External
      mask Callback PLCVarM6Scope: slplc.callbacks.updatePOUVarSS(gcb);
      mask TypeOptions PLCVarM6PortType: Hidden | Inport | Outport
      mask Callback PLCVarM6PortType: slplc.callbacks.updatePOUVarSS(gcb);
      mask TypeOptions PLCVarM6PortIndex: 1 | 2 | 3 | 4 | 5 | 6 | 7 | 8 | 9 | 10 | 11 | 12 | 13 | 14 | 15 | 16 | 17 | 18 | 19 | 20
      mask TypeOptions PLCVarM7Scope: Local | External
      mask Callback PLCVarM7Scope: slplc.callbacks.updatePOUVarSS(gcb);
      mask TypeOptions PLCVarM7PortType: Hidden | Inport | Outport
      mask Callback PLCVarM7PortType: slplc.callbacks.updatePOUVarSS(gcb);
      mask TypeOptions PLCVarM7PortIndex: 1 | 2 | 3 | 4 | 5 | 6 | 7 | 8 | 9 | 10 | 11 | 12 | 13 | 14 | 15 | 16 | 17 | 18 | 19 | 20
      mask TypeOptions PLCVarRunningScope: Local | External
      mask Callback PLCVarRunningScope: slplc.callbacks.updatePOUVarSS(gcb);
      mask TypeOptions PLCVarRunningPortType: Hidden | Inport | Outport
      mask Callback PLCVarRunningPortType: slplc.callbacks.updatePOUVarSS(gcb);
      mask TypeOptions PLCVarRunningPortIndex: 1 | 2 | 3 | 4 | 5 | 6 | 7 | 8 | 9 | 10 | 11 | 12 | 13 | 14 | 15 | 16 | 17 | 18 | 19 | 20
      mask TypeOptions PLCVarT1Scope: Local | External
      mask Callback PLCVarT1Scope: slplc.callbacks.updatePOUVarSS(gcb);
      mask TypeOptions PLCVarT1PortType: Hidden | Inport | Outport
      mask Callback PLCVarT1PortType: slplc.callbacks.updatePOUVarSS(gcb);
      mask TypeOptions PLCVarT1PortIndex: 1 | 2 | 3 | 4 | 5 | 6 | 7 | 8 | 9 | 10 | 11 | 12 | 13 | 14 | 15 | 16 | 17 | 18 | 19 | 20
      mask TypeOptions PLCVarIV1_SignalScope: Local | External
      mask Callback PLCVarIV1_SignalScope: slplc.callbacks.updatePOUVarSS(gcb);
      mask TypeOptions PLCVarIV1_SignalPortType: Hidden | Inport | Outport
      mask Callback PLCVarIV1_SignalPortType: slplc.callbacks.updatePOUVarSS(gcb);
      mask TypeOptions PLCVarIV1_SignalPortIndex: 1 | 2 | 3 | 4 | 5 | 6 | 7 | 8 | 9 | 10 | 11 | 12 | 13 | 14 | 15 | 16 | 17 | 18 | 19 | 20
      mask TypeOptions PLCVarIV2_SignalScope: Local | External
      mask Callback PLCVarIV2_SignalScope: slplc.callbacks.updatePOUVarSS(gcb);
      mask TypeOptions PLCVarIV2_SignalPortType: Hidden | Inport | Outport
      mask Callback PLCVarIV2_SignalPortType: slplc.callbacks.updatePOUVarSS(gcb);
      mask TypeOptions PLCVarIV2_SignalPortIndex: 1 | 2 | 3 | 4 | 5 | 6 | 7 | 8 | 9 | 10 | 11 | 12 | 13 | 14 | 15 | 16 | 17 | 18 | 19 | 20
      mask TypeOptions PLCVarIV3_SignalScope: Local | External
      mask Callback PLCVarIV3_SignalScope: slplc.callbacks.updatePOUVarSS(gcb);
      mask TypeOptions PLCVarIV3_SignalPortType: Hidden | Inport | Outport
      mask Callback PLCVarIV3_SignalPortType: slplc.callbacks.updatePOUVarSS(gcb);
      mask TypeOptions PLCVarIV3_SignalPortIndex: 1 | 2 | 3 | 4 | 5 | 6 | 7 | 8 | 9 | 10 | 11 | 12 | 13 | 14 | 15 | 16 | 17 | 18 | 19 | 20
      mask TypeOptions PLCVarIV4_SignalScope: Local | External
      mask Callback PLCVarIV4_SignalScope: slplc.callbacks.updatePOUVarSS(gcb);
      mask TypeOptions PLCVarIV4_SignalPortType: Hidden | Inport | Outport
      mask Callback PLCVarIV4_SignalPortType: slplc.callbacks.updatePOUVarSS(gcb);
      mask TypeOptions PLCVarIV4_SignalPortIndex: 1 | 2 | 3 | 4 | 5 | 6 | 7 | 8 | 9 | 10 | 11 | 12 | 13 | 14 | 15 | 16 | 17 | 18 | 19 | 20
      mask TypeOptions PLCVarOV_SignalScope: Local | External
      mask Callback PLCVarOV_SignalScope: slplc.callbacks.updatePOUVarSS(gcb);
      mask TypeOptions PLCVarOV_SignalPortType: Hidden | Inport | Outport
      mask Callback PLCVarOV_SignalPortType: slplc.callbacks.updatePOUVarSS(gcb);
      mask TypeOptions PLCVarOV_SignalPortIndex: 1 | 2 | 3 | 4 | 5 | 6 | 7 | 8 | 9 | 10 | 11 | 12 | 13 | 14 | 15 | 16 | 17 | 18 | 19 | 20
      mask TypeOptions PLCVarStart_ButtonScope: Local | External
      mask Callback PLCVarStart_ButtonScope: slplc.callbacks.updatePOUVarSS(gcb);
      mask TypeOptions PLCVarStart_ButtonPortType: Hidden | Inport | Outport
      mask Callback PLCVarStart_ButtonPortType: slplc.callbacks.updatePOUVarSS(gcb);
      mask TypeOptions PLCVarStart_ButtonPortIndex: 1 | 2 | 3 | 4 | 5 | 6 | 7 | 8 | 9 | 10 | 11 | 12 | 13 | 14 | 15 | 16 | 17 | 18 | 19 | 20
      mask TypeOptions PLCVarStirrer_SignalScope: Local | External
      mask Callback PLCVarStirrer_SignalScope: slplc.callbacks.updatePOUVarSS(gcb);
      mask TypeOptions PLCVarStirrer_SignalPortType: Hidden | Inport | Outport
      mask Callback PLCVarStirrer_SignalPortType: slplc.callbacks.updatePOUVarSS(gcb);
      mask TypeOptions PLCVarStirrer_SignalPortIndex: 1 | 2 | 3 | 4 | 5 | 6 | 7 | 8 | 9 | 10 | 11 | 12 | 13 | 14 | 15 | 16 | 17 | 18 | 19 | 20
      mask TypeOptions PLCVarTank_LevelScope: Local | External
      mask Callback PLCVarTank_LevelScope: slplc.callbacks.updatePOUVarSS(gcb);
      mask TypeOptions PLCVarTank_LevelPortType: Hidden | Inport | Outport
      mask Callback PLCVarTank_LevelPortType: slplc.callbacks.updatePOUVarSS(gcb);
      mask TypeOptions PLCVarTank_LevelPortIndex: 1 | 2 | 3 | 4 | 5 | 6 | 7 | 8 | 9 | 10 | 11 | 12 | 13 | 14 | 15 | 16 | 17 | 18 | 19 | 20
      mask DialogControl PLCBlockTitle Prompt: Program Variable Spreadsheet
      mask DialogControl PLCVarListHeaderName Prompt: Name
      mask DialogControl PLCVarListHeaderScope Prompt: Scope
      mask DialogControl PLCVarListHeaderDataType Prompt: Data Type
      mask DialogControl PLCVarListHeaderSize Prompt: Size
      mask DialogControl PLCVarListHeaderInitialValue Prompt: Initial Value
      mask DialogControl PLCVarListHeaderToDelete Prompt: Delete
  RES : Subsystem  Tag=B  Priority=117  TreatAsAtomicUnit=on  mask{PLCOperandTag=C1, PLCTagDataType=COUNTER, PLCBlockType=RES, PLCPOUType=stdFC, PLCOperandExpression=xxx_PLC_VAR_C1}
      mask prompts: PLCOperandTag "Operand Tag To Reset:"; PLCTagDataType "Tag Structure:"
      mask init:
      | block = gcb;
      | maskObj = Simulink.Mask.get(block);
      | maskObj.Display = sprintf('disp([''%s''  newline newline ''%s'']);', 'RES', PLCOperandTag);
      | slplc.callbacks.initResetBlock(block);
      | slplc.callbacks.initInstruction(block);
      settings: AttributesFormatString=%<PLCBlockType>: %<PLCOperandTag>
      mask Help: web([docroot '/plccoder/ref/res' '.html']);
      mask TypeOptions PLCTagDataType: TIMER | COUNTER | CONTROL
      mask DialogControl PLCBlockTitle Prompt: Reset TIMER, COUNTER, or CONTROL structure (RES)
      mask Display: disp(['RES'  newline newline 'C1']);
  RES1 : Subsystem  Tag=B  Priority=111  TreatAsAtomicUnit=on  mask{PLCOperandTag=T1, PLCTagDataType=TIMER, PLCBlockType=RES, PLCPOUType=stdFC, PLCOperandExpression=xxx_PLC_VAR_T1}
      mask prompts: PLCOperandTag "Operand Tag To Reset:"; PLCTagDataType "Tag Structure:"
      mask init: same as blending_tank_auto/PLC Controller/__Logic/Task/Program/__Logic/RES
      settings: AttributesFormatString=%<PLCBlockType>: %<PLCOperandTag>
      mask Help: web([docroot '/plccoder/ref/res' '.html']);
      mask TypeOptions PLCTagDataType: TIMER | COUNTER | CONTROL
      mask DialogControl PLCBlockTitle Prompt: Reset TIMER, COUNTER, or CONTROL structure (RES)
      mask Display: disp(['RES'  newline newline 'T1']);
  Rung Terminal : Subsystem  Priority=21  DisableCoverage=on  TreatAsAtomicUnit=on  mask{PLCRungTerminalIndex=2, PLCBlockType=RungTerminal}
      settings: AttributesFormatString=Rung %<PLCRungTerminalIndex>
      mask Help: web([docroot '/plccoder/ref/rungterminal' '.html']);
      mask DialogControl PLCBlockTitle Prompt: Rung Terminal
      mask DialogControl PLCBlockDescText Prompt: This is the ladder diagram rung terminal.
  Rung Terminal1 : Subsystem  Priority=4  DisableCoverage=on  TreatAsAtomicUnit=on  mask{PLCRungTerminalIndex=1, PLCBlockType=RungTerminal}
      settings: AttributesFormatString=Rung %<PLCRungTerminalIndex>
      mask Help: web([docroot '/plccoder/ref/rungterminal' '.html']);
      mask DialogControl PLCBlockTitle Prompt: Rung Terminal
      mask DialogControl PLCBlockDescText Prompt: This is the ladder diagram rung terminal.
  Rung Terminal10 : Subsystem  Priority=76  DisableCoverage=on  TreatAsAtomicUnit=on  mask{PLCRungTerminalIndex=10, PLCBlockType=RungTerminal}
      settings: AttributesFormatString=Rung %<PLCRungTerminalIndex>
      mask Help: web([docroot '/plccoder/ref/rungterminal' '.html']);
      mask DialogControl PLCBlockTitle Prompt: Rung Terminal
      mask DialogControl PLCBlockDescText Prompt: This is the ladder diagram rung terminal.
  Rung Terminal11 : Subsystem  Priority=82  DisableCoverage=on  TreatAsAtomicUnit=on  mask{PLCRungTerminalIndex=11, PLCBlockType=RungTerminal}
      settings: AttributesFormatString=Rung %<PLCRungTerminalIndex>
      mask Help: web([docroot '/plccoder/ref/rungterminal' '.html']);
      mask DialogControl PLCBlockTitle Prompt: Rung Terminal
      mask DialogControl PLCBlockDescText Prompt: This is the ladder diagram rung terminal.
  Rung Terminal12 : Subsystem  Priority=88  DisableCoverage=on  TreatAsAtomicUnit=on  mask{PLCRungTerminalIndex=12, PLCBlockType=RungTerminal}
      settings: AttributesFormatString=Rung %<PLCRungTerminalIndex>
      mask Help: web([docroot '/plccoder/ref/rungterminal' '.html']);
      mask DialogControl PLCBlockTitle Prompt: Rung Terminal
      mask DialogControl PLCBlockDescText Prompt: This is the ladder diagram rung terminal.
  Rung Terminal13 : Subsystem  Priority=91  DisableCoverage=on  TreatAsAtomicUnit=on  mask{PLCRungTerminalIndex=13, PLCBlockType=RungTerminal}
      settings: AttributesFormatString=Rung %<PLCRungTerminalIndex>
      mask Help: web([docroot '/plccoder/ref/rungterminal' '.html']);
      mask DialogControl PLCBlockTitle Prompt: Rung Terminal
      mask DialogControl PLCBlockDescText Prompt: This is the ladder diagram rung terminal.
  Rung Terminal14 : Subsystem  Priority=103  DisableCoverage=on  TreatAsAtomicUnit=on  mask{PLCRungTerminalIndex=17, PLCBlockType=RungTerminal}
      settings: AttributesFormatString=Rung %<PLCRungTerminalIndex>
      mask Help: web([docroot '/plccoder/ref/rungterminal' '.html']);
      mask DialogControl PLCBlockTitle Prompt: Rung Terminal
      mask DialogControl PLCBlockDescText Prompt: This is the ladder diagram rung terminal.
  Rung Terminal15 : Subsystem  Priority=94  DisableCoverage=on  TreatAsAtomicUnit=on  mask{PLCRungTerminalIndex=14, PLCBlockType=RungTerminal}
      settings: AttributesFormatString=Rung %<PLCRungTerminalIndex>
      mask Help: web([docroot '/plccoder/ref/rungterminal' '.html']);
      mask DialogControl PLCBlockTitle Prompt: Rung Terminal
      mask DialogControl PLCBlockDescText Prompt: This is the ladder diagram rung terminal.
  Rung Terminal16 : Subsystem  Priority=97  DisableCoverage=on  TreatAsAtomicUnit=on  mask{PLCRungTerminalIndex=15, PLCBlockType=RungTerminal}
      settings: AttributesFormatString=Rung %<PLCRungTerminalIndex>
      mask Help: web([docroot '/plccoder/ref/rungterminal' '.html']);
      mask DialogControl PLCBlockTitle Prompt: Rung Terminal
      mask DialogControl PLCBlockDescText Prompt: This is the ladder diagram rung terminal.
  Rung Terminal17 : Subsystem  Priority=100  DisableCoverage=on  TreatAsAtomicUnit=on  mask{PLCRungTerminalIndex=16, PLCBlockType=RungTerminal}
      settings: AttributesFormatString=Rung %<PLCRungTerminalIndex>
      mask Help: web([docroot '/plccoder/ref/rungterminal' '.html']);
      mask DialogControl PLCBlockTitle Prompt: Rung Terminal
      mask DialogControl PLCBlockDescText Prompt: This is the ladder diagram rung terminal.
  Rung Terminal18 : Subsystem  Priority=109  DisableCoverage=on  TreatAsAtomicUnit=on  mask{PLCRungTerminalIndex=19, PLCBlockType=RungTerminal}
      settings: AttributesFormatString=Rung %<PLCRungTerminalIndex>
      mask Help: web([docroot '/plccoder/ref/rungterminal' '.html']);
      mask DialogControl PLCBlockTitle Prompt: Rung Terminal
      mask DialogControl PLCBlockDescText Prompt: This is the ladder diagram rung terminal.
  Rung Terminal19 : Subsystem  Priority=112  DisableCoverage=on  TreatAsAtomicUnit=on  mask{PLCRungTerminalIndex=20, PLCBlockType=RungTerminal}
      settings: AttributesFormatString=Rung %<PLCRungTerminalIndex>
      mask Help: web([docroot '/plccoder/ref/rungterminal' '.html']);
      mask DialogControl PLCBlockTitle Prompt: Rung Terminal
      mask DialogControl PLCBlockDescText Prompt: This is the ladder diagram rung terminal.
  Rung Terminal2 : Subsystem  Priority=24  DisableCoverage=on  TreatAsAtomicUnit=on  mask{PLCRungTerminalIndex=3, PLCBlockType=RungTerminal}
      settings: AttributesFormatString=Rung %<PLCRungTerminalIndex>
      mask Help: web([docroot '/plccoder/ref/rungterminal' '.html']);
      mask DialogControl PLCBlockTitle Prompt: Rung Terminal
      mask DialogControl PLCBlockDescText Prompt: This is the ladder diagram rung terminal.
  Rung Terminal20 : Subsystem  Priority=115  DisableCoverage=on  TreatAsAtomicUnit=on  mask{PLCRungTerminalIndex=21, PLCBlockType=RungTerminal}
      settings: AttributesFormatString=Rung %<PLCRungTerminalIndex>
      mask Help: web([docroot '/plccoder/ref/rungterminal' '.html']);
      mask DialogControl PLCBlockTitle Prompt: Rung Terminal
      mask DialogControl PLCBlockDescText Prompt: This is the ladder diagram rung terminal.
  Rung Terminal21 : Subsystem  Priority=118  DisableCoverage=on  TreatAsAtomicUnit=on  mask{PLCRungTerminalIndex=22, PLCBlockType=RungTerminal}
      settings: AttributesFormatString=Rung %<PLCRungTerminalIndex>
      mask Help: web([docroot '/plccoder/ref/rungterminal' '.html']);
      mask DialogControl PLCBlockTitle Prompt: Rung Terminal
      mask DialogControl PLCBlockDescText Prompt: This is the ladder diagram rung terminal.
  Rung Terminal3 : Subsystem  Priority=30  DisableCoverage=on  TreatAsAtomicUnit=on  mask{PLCRungTerminalIndex=4, PLCBlockType=RungTerminal}
      settings: AttributesFormatString=Rung %<PLCRungTerminalIndex>
      mask Help: web([docroot '/plccoder/ref/rungterminal' '.html']);
      mask DialogControl PLCBlockTitle Prompt: Rung Terminal
      mask DialogControl PLCBlockDescText Prompt: This is the ladder diagram rung terminal.
  Rung Terminal4 : Subsystem  Priority=38  DisableCoverage=on  TreatAsAtomicUnit=on  mask{PLCRungTerminalIndex=5, PLCBlockType=RungTerminal}
      settings: AttributesFormatString=Rung %<PLCRungTerminalIndex>
      mask Help: web([docroot '/plccoder/ref/rungterminal' '.html']);
      mask DialogControl PLCBlockTitle Prompt: Rung Terminal
      mask DialogControl PLCBlockDescText Prompt: This is the ladder diagram rung terminal.
  Rung Terminal5 : Subsystem  Priority=46  DisableCoverage=on  TreatAsAtomicUnit=on  mask{PLCRungTerminalIndex=6, PLCBlockType=RungTerminal}
      settings: AttributesFormatString=Rung %<PLCRungTerminalIndex>
      mask Help: web([docroot '/plccoder/ref/rungterminal' '.html']);
      mask DialogControl PLCBlockTitle Prompt: Rung Terminal
      mask DialogControl PLCBlockDescText Prompt: This is the ladder diagram rung terminal.
  Rung Terminal6 : Subsystem  Priority=54  DisableCoverage=on  TreatAsAtomicUnit=on  mask{PLCRungTerminalIndex=7, PLCBlockType=RungTerminal}
      settings: AttributesFormatString=Rung %<PLCRungTerminalIndex>
      mask Help: web([docroot '/plccoder/ref/rungterminal' '.html']);
      mask DialogControl PLCBlockTitle Prompt: Rung Terminal
      mask DialogControl PLCBlockDescText Prompt: This is the ladder diagram rung terminal.
  Rung Terminal7 : Subsystem  Priority=68  DisableCoverage=on  TreatAsAtomicUnit=on  mask{PLCRungTerminalIndex=9, PLCBlockType=RungTerminal}
      settings: AttributesFormatString=Rung %<PLCRungTerminalIndex>
      mask Help: web([docroot '/plccoder/ref/rungterminal' '.html']);
      mask DialogControl PLCBlockTitle Prompt: Rung Terminal
      mask DialogControl PLCBlockDescText Prompt: This is the ladder diagram rung terminal.
  Rung Terminal8 : Subsystem  Priority=62  DisableCoverage=on  TreatAsAtomicUnit=on  mask{PLCRungTerminalIndex=8, PLCBlockType=RungTerminal}
      settings: AttributesFormatString=Rung %<PLCRungTerminalIndex>
      mask Help: web([docroot '/plccoder/ref/rungterminal' '.html']);
      mask DialogControl PLCBlockTitle Prompt: Rung Terminal
      mask DialogControl PLCBlockDescText Prompt: This is the ladder diagram rung terminal.
  Rung Terminal9 : Subsystem  Priority=106  DisableCoverage=on  TreatAsAtomicUnit=on  mask{PLCRungTerminalIndex=18, PLCBlockType=RungTerminal}
      settings: AttributesFormatString=Rung %<PLCRungTerminalIndex>
      mask Help: web([docroot '/plccoder/ref/rungterminal' '.html']);
      mask DialogControl PLCBlockTitle Prompt: Rung Terminal
      mask DialogControl PLCBlockDescText Prompt: This is the ladder diagram rung terminal.
  TON : Subsystem  Priority=108  TreatAsAtomicUnit=on  mask{PLCOperandTag=T1, PLCTimerSampleTime=0.2, PLCBlockType=TON, PLCPOUType=stdFB, PLCOperandAccess=ReadWrite, PLCOperandExpression=xxx_PLC_VAR_T1}
      mask prompts: PLCOperandTag "Timer Tag:"; PLCTimerSampleTime "Timer Sample Time:"
      mask init:
      | block = gcb;
      | maskObj = Simulink.Mask.get(block);
      | maskObj.Display = sprintf('disp([''%s'' newline newline ''%s'']);', PLCBlockType, PLCOperandTag);
      | slplc.callbacks.initInstruction(block);
      settings: AttributesFormatString=%<PLCBlockType>: %<PLCOperandTag>
      mask Help: web([docroot '/plccoder/ref/ton' '.html']);
      mask DialogControl PLCBlockTitle Prompt: Timer On Delay (TON)
      mask Display: disp(['TON' newline newline 'T1']);
  Up to Parent POU : Subsystem  DisableCoverage=on  TreatAsAtomicUnit=on  mask{PLCBlockType=OpenParentPOU}
      settings: OpenFcn=slplc.callbacks.openParentPOUBlock(gcb);
      mask Help: web([docroot '/plccoder/ref/uptoparentpou' '.html']);
      mask DialogControl PLCBlockTitle Prompt: Add Single Rung
  Variable Read : Subsystem  Priority=33  TreatAsAtomicUnit=on  mask{PLCOperandTag=Tank_Level, PLCBlockType=VariableRead, PLCOperandAccess=Read, PLCPOUType=VariableRead, PLCOperandExpression=xxx_PLC_VAR_Tank_Level}
      mask prompts: PLCOperandTag "Data Tag:"
      mask init:
      | block = gcb;
      | maskObj = Simulink.Mask.get(block);
      | maskObj.Display = sprintf('disp(''%s'');', PLCOperandTag);
      | slplc.callbacks.initInstruction(block);
      mask Help: web([docroot '/plccoder/ref/variableread' '.html']);
      mask DialogControl PLCBlockTitle Prompt: Data Tag Read
      mask Display: disp('Tank_Level');
  Variable Read1 : Subsystem  Priority=41  TreatAsAtomicUnit=on  mask{PLCOperandTag=Tank_Level, PLCBlockType=VariableRead, PLCOperandAccess=Read, PLCPOUType=VariableRead, PLCOperandExpression=xxx_PLC_VAR_Tank_Level}
      mask prompts: PLCOperandTag "Data Tag:"
      mask init:
      | block = gcb;
      | maskObj = Simulink.Mask.get(block);
      | maskObj.Display = sprintf('disp(''%s'');', PLCOperandTag);
      | slplc.callbacks.initInstruction(block);
      mask Help: web([docroot '/plccoder/ref/variableread' '.html']);
      mask DialogControl PLCBlockTitle Prompt: Data Tag Read
      mask Display: disp('Tank_Level');
  Variable Read2 : Subsystem  Priority=49  TreatAsAtomicUnit=on  mask{PLCOperandTag=Tank_Level, PLCBlockType=VariableRead, PLCOperandAccess=Read, PLCPOUType=VariableRead, PLCOperandExpression=xxx_PLC_VAR_Tank_Level}
      mask prompts: PLCOperandTag "Data Tag:"
      mask init:
      | block = gcb;
      | maskObj = Simulink.Mask.get(block);
      | maskObj.Display = sprintf('disp(''%s'');', PLCOperandTag);
      | slplc.callbacks.initInstruction(block);
      mask Help: web([docroot '/plccoder/ref/variableread' '.html']);
      mask DialogControl PLCBlockTitle Prompt: Data Tag Read
      mask Display: disp('Tank_Level');
  Variable Read3 : Subsystem  Priority=57  TreatAsAtomicUnit=on  mask{PLCOperandTag=Tank_Level, PLCBlockType=VariableRead, PLCOperandAccess=Read, PLCPOUType=VariableRead, PLCOperandExpression=xxx_PLC_VAR_Tank_Level}
      mask prompts: PLCOperandTag "Data Tag:"
      mask init:
      | block = gcb;
      | maskObj = Simulink.Mask.get(block);
      | maskObj.Display = sprintf('disp(''%s'');', PLCOperandTag);
      | slplc.callbacks.initInstruction(block);
      mask Help: web([docroot '/plccoder/ref/variableread' '.html']);
      mask DialogControl PLCBlockTitle Prompt: Data Tag Read
      mask Display: disp('Tank_Level');
  Variable Read4 : Subsystem  Priority=71  TreatAsAtomicUnit=on  mask{PLCOperandTag=Tank_Level, PLCBlockType=VariableRead, PLCOperandAccess=Read, PLCPOUType=VariableRead, PLCOperandExpression=xxx_PLC_VAR_Tank_Level}
      mask prompts: PLCOperandTag "Data Tag:"
      mask init:
      | block = gcb;
      | maskObj = Simulink.Mask.get(block);
      | maskObj.Display = sprintf('disp(''%s'');', PLCOperandTag);
      | slplc.callbacks.initInstruction(block);
      mask Help: web([docroot '/plccoder/ref/variableread' '.html']);
      mask DialogControl PLCBlockTitle Prompt: Data Tag Read
      mask Display: disp('Tank_Level');
  XIC : Subsystem  Priority=5  TreatAsAtomicUnit=on  mask{PLCOperandTag=Initialise, PLCBlockType=XIC, PLCPOUType=Contact, PLCOperandExpression=xxx_PLC_VAR_Initialise}
      mask prompts: PLCOperandTag "Operand Tag:"
      mask init:
      | slplc.callbacks.initInstruction(gcb);
      settings: AttributesFormatString=%<PLCOperandTag>
      mask Help: web([docroot '/plccoder/ref/xic' '.html']);
      mask DialogControl PLCBlockTitle Prompt: Examine If Closed (XIC)
  XIC1 : Subsystem  Priority=25  TreatAsAtomicUnit=on  mask{PLCOperandTag=M0, PLCBlockType=XIC, PLCPOUType=Contact, PLCOperandExpression=xxx_PLC_VAR_M0}
      mask prompts: PLCOperandTag "Operand Tag:"
      mask init:
      | slplc.callbacks.initInstruction(gcb);
      settings: AttributesFormatString=%<PLCOperandTag>
      mask Help: web([docroot '/plccoder/ref/xic' '.html']);
      mask DialogControl PLCBlockTitle Prompt: Examine If Closed (XIC)
  XIC10 : Subsystem  Priority=69  TreatAsAtomicUnit=on  mask{PLCOperandTag=M6, PLCBlockType=XIC, PLCPOUType=Contact, PLCOperandExpression=xxx_PLC_VAR_M6}
      mask prompts: PLCOperandTag "Operand Tag:"
      mask init:
      | slplc.callbacks.initInstruction(gcb);
      settings: AttributesFormatString=%<PLCOperandTag>
      mask Help: web([docroot '/plccoder/ref/xic' '.html']);
      mask DialogControl PLCBlockTitle Prompt: Examine If Closed (XIC)
  XIC11 : Subsystem  Priority=77  TreatAsAtomicUnit=on  mask{PLCOperandTag=M7, PLCBlockType=XIC, PLCPOUType=Contact, PLCOperandExpression=xxx_PLC_VAR_M7}
      mask prompts: PLCOperandTag "Operand Tag:"
      mask init:
      | slplc.callbacks.initInstruction(gcb);
      settings: AttributesFormatString=%<PLCOperandTag>
      mask Help: web([docroot '/plccoder/ref/xic' '.html']);
      mask DialogControl PLCBlockTitle Prompt: Examine If Closed (XIC)
  XIC12 : Subsystem  Priority=107  TreatAsAtomicUnit=on  mask{PLCOperandTag=M5, PLCBlockType=XIC, PLCPOUType=Contact, PLCOperandExpression=xxx_PLC_VAR_M5}
      mask prompts: PLCOperandTag "Operand Tag:"
      mask init:
      | slplc.callbacks.initInstruction(gcb);
      settings: AttributesFormatString=%<PLCOperandTag>
      mask Help: web([docroot '/plccoder/ref/xic' '.html']);
      mask DialogControl PLCBlockTitle Prompt: Examine If Closed (XIC)
  XIC13 : Subsystem  Priority=89  TreatAsAtomicUnit=on  mask{PLCOperandTag=M2, PLCBlockType=XIC, PLCPOUType=Contact, PLCOperandExpression=xxx_PLC_VAR_M2}
      mask prompts: PLCOperandTag "Operand Tag:"
      mask init:
      | slplc.callbacks.initInstruction(gcb);
      settings: AttributesFormatString=%<PLCOperandTag>
      mask Help: web([docroot '/plccoder/ref/xic' '.html']);
      mask DialogControl PLCBlockTitle Prompt: Examine If Closed (XIC)
  XIC14 : Subsystem  Priority=92  TreatAsAtomicUnit=on  mask{PLCOperandTag=M3, PLCBlockType=XIC, PLCPOUType=Contact, PLCOperandExpression=xxx_PLC_VAR_M3}
      mask prompts: PLCOperandTag "Operand Tag:"
      mask init:
      | slplc.callbacks.initInstruction(gcb);
      settings: AttributesFormatString=%<PLCOperandTag>
      mask Help: web([docroot '/plccoder/ref/xic' '.html']);
      mask DialogControl PLCBlockTitle Prompt: Examine If Closed (XIC)
  XIC15 : Subsystem  Priority=95  TreatAsAtomicUnit=on  mask{PLCOperandTag=M4, PLCBlockType=XIC, PLCPOUType=Contact, PLCOperandExpression=xxx_PLC_VAR_M4}
      mask prompts: PLCOperandTag "Operand Tag:"
      mask init:
      | slplc.callbacks.initInstruction(gcb);
      settings: AttributesFormatString=%<PLCOperandTag>
      mask Help: web([docroot '/plccoder/ref/xic' '.html']);
      mask DialogControl PLCBlockTitle Prompt: Examine If Closed (XIC)
  XIC16 : Subsystem  Priority=98  TreatAsAtomicUnit=on  mask{PLCOperandTag=M1, PLCBlockType=XIC, PLCPOUType=Contact, PLCOperandExpression=xxx_PLC_VAR_M1}
      mask prompts: PLCOperandTag "Operand Tag:"
      mask init:
      | slplc.callbacks.initInstruction(gcb);
      settings: AttributesFormatString=%<PLCOperandTag>
      mask Help: web([docroot '/plccoder/ref/xic' '.html']);
      mask DialogControl PLCBlockTitle Prompt: Examine If Closed (XIC)
  XIC17 : Subsystem  Priority=101  TreatAsAtomicUnit=on  mask{PLCOperandTag=M6, PLCBlockType=XIC, PLCPOUType=Contact, PLCOperandExpression=xxx_PLC_VAR_M6}
      mask prompts: PLCOperandTag "Operand Tag:"
      mask init:
      | slplc.callbacks.initInstruction(gcb);
      settings: AttributesFormatString=%<PLCOperandTag>
      mask Help: web([docroot '/plccoder/ref/xic' '.html']);
      mask DialogControl PLCBlockTitle Prompt: Examine If Closed (XIC)
  XIC18 : Subsystem  Priority=104  TreatAsAtomicUnit=on  mask{PLCOperandTag=M5, PLCBlockType=XIC, PLCPOUType=Contact, PLCOperandExpression=xxx_PLC_VAR_M5}
      mask prompts: PLCOperandTag "Operand Tag:"
      mask init:
      | slplc.callbacks.initInstruction(gcb);
      settings: AttributesFormatString=%<PLCOperandTag>
      mask Help: web([docroot '/plccoder/ref/xic' '.html']);
      mask DialogControl PLCBlockTitle Prompt: Examine If Closed (XIC)
  XIC19 : Subsystem  Priority=113  TreatAsAtomicUnit=on  mask{PLCOperandTag=M6, PLCBlockType=XIC, PLCPOUType=Contact, PLCOperandExpression=xxx_PLC_VAR_M6}
      mask prompts: PLCOperandTag "Operand Tag:"
      mask init:
      | slplc.callbacks.initInstruction(gcb);
      settings: AttributesFormatString=%<PLCOperandTag>
      mask Help: web([docroot '/plccoder/ref/xic' '.html']);
      mask DialogControl PLCBlockTitle Prompt: Examine If Closed (XIC)
  XIC2 : Subsystem  Priority=26  TreatAsAtomicUnit=on  mask{PLCOperandTag=Start_Button, PLCBlockType=XIC, PLCPOUType=Contact, PLCOperandExpression=xxx_PLC_VAR_Start_Button}
      mask prompts: PLCOperandTag "Operand Tag:"
      mask init:
      | slplc.callbacks.initInstruction(gcb);
      settings: AttributesFormatString=%<PLCOperandTag>
      mask Help: web([docroot '/plccoder/ref/xic' '.html']);
      mask DialogControl PLCBlockTitle Prompt: Examine If Closed (XIC)
  XIC20 : Subsystem  Priority=83  TreatAsAtomicUnit=on  mask{PLCOperandTag=M7, PLCBlockType=XIC, PLCPOUType=Contact, PLCOperandExpression=xxx_PLC_VAR_M7}
      mask prompts: PLCOperandTag "Operand Tag:"
      mask init:
      | slplc.callbacks.initInstruction(gcb);
      settings: AttributesFormatString=%<PLCOperandTag>
      mask Help: web([docroot '/plccoder/ref/xic' '.html']);
      mask DialogControl PLCBlockTitle Prompt: Examine If Closed (XIC)
  XIC21 : Subsystem  Priority=84  TreatAsAtomicUnit=on  mask{PLCOperandTag=C1.DN, PLCBlockType=XIC, PLCPOUType=Contact, PLCOperandExpression=xxx_PLC_VAR_C1.DN}
      mask prompts: PLCOperandTag "Operand Tag:"
      mask init:
      | slplc.callbacks.initInstruction(gcb);
      settings: AttributesFormatString=%<PLCOperandTag>
      mask Help: web([docroot '/plccoder/ref/xic' '.html']);
      mask DialogControl PLCBlockTitle Prompt: Examine If Closed (XIC)
  XIC22 : Subsystem  Priority=116  TreatAsAtomicUnit=on  mask{PLCOperandTag=M0, PLCBlockType=XIC, PLCPOUType=Contact, PLCOperandExpression=xxx_PLC_VAR_M0}
      mask prompts: PLCOperandTag "Operand Tag:"
      mask init:
      | slplc.callbacks.initInstruction(gcb);
      settings: AttributesFormatString=%<PLCOperandTag>
      mask Help: web([docroot '/plccoder/ref/xic' '.html']);
      mask DialogControl PLCBlockTitle Prompt: Examine If Closed (XIC)
  XIC23 : Subsystem  Priority=110  TreatAsAtomicUnit=on  mask{PLCOperandTag=M1, PLCBlockType=XIC, PLCPOUType=Contact, PLCOperandExpression=xxx_PLC_VAR_M1}
      mask prompts: PLCOperandTag "Operand Tag:"
      mask init:
      | slplc.callbacks.initInstruction(gcb);
      settings: AttributesFormatString=%<PLCOperandTag>
      mask Help: web([docroot '/plccoder/ref/xic' '.html']);
      mask DialogControl PLCBlockTitle Prompt: Examine If Closed (XIC)
  XIC3 : Subsystem  Priority=31  TreatAsAtomicUnit=on  mask{PLCOperandTag=M1, PLCBlockType=XIC, PLCPOUType=Contact, PLCOperandExpression=xxx_PLC_VAR_M1}
      mask prompts: PLCOperandTag "Operand Tag:"
      mask init:
      | slplc.callbacks.initInstruction(gcb);
      settings: AttributesFormatString=%<PLCOperandTag>
      mask Help: web([docroot '/plccoder/ref/xic' '.html']);
      mask DialogControl PLCBlockTitle Prompt: Examine If Closed (XIC)
  XIC4 : Subsystem  Priority=39  TreatAsAtomicUnit=on  mask{PLCOperandTag=M2, PLCBlockType=XIC, PLCPOUType=Contact, PLCOperandExpression=xxx_PLC_VAR_M2}
      mask prompts: PLCOperandTag "Operand Tag:"
      mask init:
      | slplc.callbacks.initInstruction(gcb);
      settings: AttributesFormatString=%<PLCOperandTag>
      mask Help: web([docroot '/plccoder/ref/xic' '.html']);
      mask DialogControl PLCBlockTitle Prompt: Examine If Closed (XIC)
  XIC5 : Subsystem  Priority=47  TreatAsAtomicUnit=on  mask{PLCOperandTag=M3, PLCBlockType=XIC, PLCPOUType=Contact, PLCOperandExpression=xxx_PLC_VAR_M3}
      mask prompts: PLCOperandTag "Operand Tag:"
      mask init:
      | slplc.callbacks.initInstruction(gcb);
      settings: AttributesFormatString=%<PLCOperandTag>
      mask Help: web([docroot '/plccoder/ref/xic' '.html']);
      mask DialogControl PLCBlockTitle Prompt: Examine If Closed (XIC)
  XIC6 : Subsystem  Priority=55  TreatAsAtomicUnit=on  mask{PLCOperandTag=M4, PLCBlockType=XIC, PLCPOUType=Contact, PLCOperandExpression=xxx_PLC_VAR_M4}
      mask prompts: PLCOperandTag "Operand Tag:"
      mask init:
      | slplc.callbacks.initInstruction(gcb);
      settings: AttributesFormatString=%<PLCOperandTag>
      mask Help: web([docroot '/plccoder/ref/xic' '.html']);
      mask DialogControl PLCBlockTitle Prompt: Examine If Closed (XIC)
  XIC7 : Subsystem  Priority=63  TreatAsAtomicUnit=on  mask{PLCOperandTag=M5, PLCBlockType=XIC, PLCPOUType=Contact, PLCOperandExpression=xxx_PLC_VAR_M5}
      mask prompts: PLCOperandTag "Operand Tag:"
      mask init:
      | slplc.callbacks.initInstruction(gcb);
      settings: AttributesFormatString=%<PLCOperandTag>
      mask Help: web([docroot '/plccoder/ref/xic' '.html']);
      mask DialogControl PLCBlockTitle Prompt: Examine If Closed (XIC)
  XIC8 : Subsystem  Priority=64  TreatAsAtomicUnit=on  mask{PLCOperandTag=T1.DN, PLCBlockType=XIC, PLCPOUType=Contact, PLCOperandExpression=xxx_PLC_VAR_T1.DN}
      mask prompts: PLCOperandTag "Operand Tag:"
      mask init:
      | slplc.callbacks.initInstruction(gcb);
      settings: AttributesFormatString=%<PLCOperandTag>
      mask Help: web([docroot '/plccoder/ref/xic' '.html']);
      mask DialogControl PLCBlockTitle Prompt: Examine If Closed (XIC)
  XIC9 : Subsystem  Priority=22  TreatAsAtomicUnit=on  mask{PLCOperandTag=Initialise, PLCBlockType=XIC, PLCPOUType=Contact, PLCOperandExpression=xxx_PLC_VAR_Initialise}
      mask prompts: PLCOperandTag "Operand Tag:"
      mask init:
      | slplc.callbacks.initInstruction(gcb);
      settings: AttributesFormatString=%<PLCOperandTag>
      mask Help: web([docroot '/plccoder/ref/xic' '.html']);
      mask DialogControl PLCBlockTitle Prompt: Examine If Closed (XIC)
  XIO : Subsystem  Priority=2  TreatAsAtomicUnit=on  mask{PLCOperandExpression=xxx_PLC_VAR_Running, PLCOperandTag=Running, PLCBlockType=XIO, PLCPOUType=Contact}
      mask prompts: PLCOperandTag "Operand Tag:"
      mask init:
      | slplc.callbacks.initInstruction(gcb);
      settings: AttributesFormatString=%<PLCOperandTag>
      mask Help: web([docroot '/plccoder/ref/xio' '.html']);
      mask DialogControl PLCBlockTitle Prompt: Examine If Open (XIO)
  XIO1 : Subsystem  Priority=78  TreatAsAtomicUnit=on  mask{PLCOperandExpression=xxx_PLC_VAR_C1.DN, PLCOperandTag=C1.DN, PLCBlockType=XIO, PLCPOUType=Contact}
      mask prompts: PLCOperandTag "Operand Tag:"
      mask init:
      | slplc.callbacks.initInstruction(gcb);
      settings: AttributesFormatString=%<PLCOperandTag>
      mask Help: web([docroot '/plccoder/ref/xio' '.html']);
      mask DialogControl PLCBlockTitle Prompt: Examine If Open (XIO)
  wires:
  OTL6/1(RungOut) -> Rung Terminal2/1(RungIn)
  XIC9/1(RungOut) -> OTL6/1(RungIn)
  OTE/1(RungOut) -> Rung Terminal1/1(RungIn)
  XIC/1(RungOut) -> OTU15/1(RungIn), OTU14/1(RungIn), OTU13/1(RungIn), OTU12/1(RungIn), OTU11/1(RungIn), OTU10/1(RungIn), OTU/1(RungIn), OTL/1(RungIn)
  XIO/1(RungOut) -> OTE/1(RungIn)
  Junction1/1(RungOut) -> Rung Terminal3/1(RungIn)
  OTU1/1(RungOut) -> Junction1/2(RungIn2)
  XIC1/1(RungOut) -> XIC2/1(RungIn)
  OTL2/1(RungOut) -> Junction1/1(RungIn1)
  XIC2/1(RungOut) -> OTU1/1(RungIn), OTL2/1(RungIn)
  XIC3/1(RungOut) -> LEQ_1/1(RungIn)
  Variable Read/1(VarOut) -> LEQ_1/3(srcB)
  Constant/1 -> LEQ_1/2(srcA)
  Junction2/1(RungOut) -> Rung Terminal4/1(RungIn)
  OTL1/1(RungOut) -> Junction2/1(RungIn1)
  OTU2/1(RungOut) -> Junction2/2(RungIn2)
  LEQ_1/1(RungOut) -> OTU2/1(RungIn), OTL1/1(RungIn)
  OTU3/1(RungOut) -> Junction3/2(RungIn2)
  Variable Read1/1(VarOut) -> LEQ_2/3(srcB)
  Constant1/1 -> LEQ_2/2(srcA)
  XIC4/1(RungOut) -> LEQ_2/1(RungIn)
  LEQ_2/1(RungOut) -> OTU3/1(RungIn), OTL3/1(RungIn)
  OTL3/1(RungOut) -> Junction3/1(RungIn1)
  Junction3/1(RungOut) -> Rung Terminal5/1(RungIn)
  OTL4/1(RungOut) -> Junction4/1(RungIn1)
  LEQ_3/1(RungOut) -> OTU4/1(RungIn), OTL4/1(RungIn)
  OTU4/1(RungOut) -> Junction4/2(RungIn2)
  Constant2/1 -> LEQ_3/2(srcA)
  Junction4/1(RungOut) -> Rung Terminal6/1(RungIn)
  Variable Read2/1(VarOut) -> LEQ_3/3(srcB)
  XIC5/1(RungOut) -> LEQ_3/1(RungIn)
  Variable Read3/1(VarOut) -> LEQ_4/3(srcB)
  Constant3/1 -> LEQ_4/2(srcA)
  XIC6/1(RungOut) -> LEQ_4/1(RungIn)
  Junction5/1(RungOut) -> Rung Terminal8/1(RungIn)
  OTU5/1(RungOut) -> Junction5/2(RungIn2)
  LEQ_4/1(RungOut) -> OTU5/1(RungIn), OTL5/1(RungIn)
  OTL5/1(RungOut) -> Junction5/1(RungIn1)
  XIC7/1(RungOut) -> XIC8/1(RungIn)
  OTU6/1(RungOut) -> Junction6/2(RungIn2)
  XIC8/1(RungOut) -> OTU6/1(RungIn), OTL7/1(RungIn)
  OTL7/1(RungOut) -> Junction6/1(RungIn1)
  Junction6/1(RungOut) -> Rung Terminal7/1(RungIn)
  OTL8/1(RungOut) -> Junction7/1(RungIn1)
  EQU/1(RungOut) -> OTU7/1(RungIn), OTL8/1(RungIn)
  Junction7/1(RungOut) -> Rung Terminal10/1(RungIn)
  XIC10/1(RungOut) -> EQU/1(RungIn)
  OTU7/1(RungOut) -> Junction7/2(RungIn2)
  Constant4/1 -> EQU/2(srcA)
  Variable Read4/1(VarOut) -> EQU/3(srcB)
  XIC11/1(RungOut) -> XIO1/1(RungIn)
  TON/1(EN) -> Rung Terminal18/1(RungIn)
  XIC12/1(RungOut) -> TON/1(RungIn)
  XIC18/1(RungOut) -> OTE6/1(RungIn)
  OTE6/1(RungOut) -> Rung Terminal9/1(RungIn)
  XIC17/1(RungOut) -> OTE5/1(RungIn)
  OTE5/1(RungOut) -> Rung Terminal14/1(RungIn)
  OTE4/1(RungOut) -> Rung Terminal17/1(RungIn)
  XIC16/1(RungOut) -> OTE4/1(RungIn)
  OTE3/1(RungOut) -> Rung Terminal16/1(RungIn)
  XIC15/1(RungOut) -> OTE3/1(RungIn)
  XIC14/1(RungOut) -> OTE2/1(RungIn)
  OTE2/1(RungOut) -> Rung Terminal15/1(RungIn)
  OTU9/1(RungOut) -> Junction9/2(RungIn2)
  OTL10/1(RungOut) -> Junction9/1(RungIn1)
  XIC21/1(RungOut) -> OTU9/1(RungIn), OTL10/1(RungIn)
  Power Rail Start/1(PowerOut) -> XIC23/1(RungIn), XIC19/1(RungIn), XIC22/1(RungIn), Power Rail Terminal/1(PowerIn), XIC12/1(RungIn), XIC18/1(RungIn), XIC17/1(RungIn), XIC16/1(RungIn), XIC15/1(RungIn), XIC14/1(RungIn), XIC13/1(RungIn), XIC20/1(RungIn), XIC11/1(RungIn), XIC10/1(RungIn), XIC7/1(RungIn), XIC6/1(RungIn), XIC5/1(RungIn), XIC4/1(RungIn), XIC3/1(RungIn), XIC1/1(RungIn), XIC9/1(RungIn), XIC/1(RungIn), XIO/1(RungIn)
  OTU8/1(RungOut) -> Junction8/2(RungIn2)
  OTL9/1(RungOut) -> Junction8/1(RungIn1)
  XIO1/1(RungOut) -> OTU8/1(RungIn), OTL9/1(RungIn)
  Junction8/1(RungOut) -> Rung Terminal11/1(RungIn)
  Junction9/1(RungOut) -> Rung Terminal12/1(RungIn)
  XIC20/1(RungOut) -> XIC21/1(RungIn)
  XIC13/1(RungOut) -> OTE1/1(RungIn)
  OTE1/1(RungOut) -> Rung Terminal13/1(RungIn)
  RES/1(RungOut) -> Rung Terminal21/1(RungIn)
  XIC22/1(RungOut) -> RES/1(RungIn)
  XIC19/1(RungOut) -> CTU/1(RungIn)
  CTU/1(CU) -> Rung Terminal20/1(RungIn)
  RES1/1(RungOut) -> Rung Terminal19/1(RungIn)
  XIC23/1(RungOut) -> RES1/1(RungIn)
  OTU14/1(RungOut) -> Junction10/1(RungIn1)
  OTU15/1(RungOut) -> Junction10/2(RungIn2)
  Junction10/1(RungOut) -> Junction11/2(RungIn2)
  OTU13/1(RungOut) -> Junction11/1(RungIn1)
  OTU11/1(RungOut) -> Junction13/1(RungIn1)
  Junction12/1(RungOut) -> Junction13/2(RungIn2)
  Junction11/1(RungOut) -> Junction12/2(RungIn2)
  OTU12/1(RungOut) -> Junction12/1(RungIn1)
  OTU10/1(RungOut) -> Junction15/1(RungIn1)
  OTU/1(RungOut) -> Junction16/1(RungIn1)
  OTL/1(RungOut) -> Junction17/1(RungIn1)
  Junction15/1(RungOut) -> Junction16/2(RungIn2)
  Junction16/1(RungOut) -> Junction17/2(RungIn2)
  Junction13/1(RungOut) -> Junction15/2(RungIn2)
  Junction17/1(RungOut) -> Rung Terminal/1(RungIn)
